simulink model "TrialMBD"  (R2021a)
settings: Solver=FixedStepDiscrete  StartTime=0.0  StopTime=10.0  RelTol=1e-3
libraries: simulink x2
settings Model: Creator=Mahmoud Sofar  LastModifiedBy=Mahmoud Sofar
settings OptimizationCC: DefaultParameterBehavior=Inlined  EnhancedBackFolding=on  PassReuseOutputArgsAs=Individual arguments  ZeroExternalMemoryAtStartup=off  ZeroInternalMemoryAtStartup=off  OptimizeBlockOrder=speed  DifferentSizesBufferReuse=on  OptimizationCustomize=off  EfficientTunableParamExpr=on
settings DebuggingCC: ParameterTunabilityLossMsg=error
settings SFSimCC: MATLABDynamicMemAlloc=off
settings RTWCC: SystemTargetFile=ert.tlc  GenCodeOnly=on  TemplateMakefile=ert_default_tmf  GenerateReport=on  IncludeHyperlinkInReport=on  LaunchReport=on  GenerateTraceInfo=on
settings CodeAppCC: ForceParamTrailComments=on  IgnoreCustomStorageClasses=off  OperatorAnnotations=on  SimulinkDataObjDesc=on  SFDataObjDesc=on  InsertBlockDesc=on
settings ERTTargetCC: TargetLangStandard=C99 (ISO)  GenerateSampleERTMain=on  InlinedParameterPlacement=NonHierarchical  ERTCustomFileTemplate=example_file_process.tlc

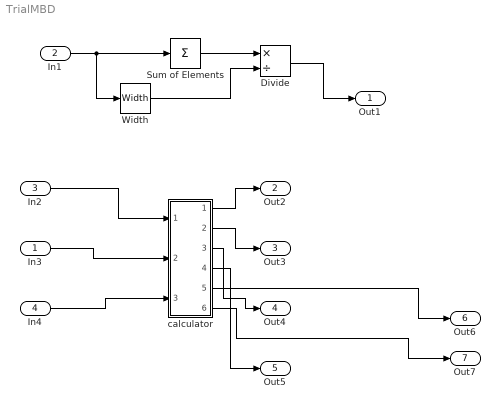
== system TrialMBD ==
  In3 : Inport  PortDimensions=1
  In1 : Inport  Port=2  PortDimensions=11
  In2 : Inport  Port=3  PortDimensions=1
  In4 : Inport  Port=4  PortDimensions=1
  Divide : Product  Inputs=*/
  Sum of Elements : Sum  Inputs=+
  Width : Width
  calculator : Subsystem
  Out1 : Outport
  Out2 : Outport  Port=2
  Out3 : Outport  Port=3
  Out4 : Outport  Port=4
  Out5 : Outport  Port=5
  Out6 : Outport  Port=6
  Out7 : Outport  Port=7
  wires:
  In1/1 -> Width/1, Sum of Elements/1
  Sum of Elements/1 -> Divide/1
  Divide/1 -> Out1/1
  Width/1 -> Divide/2
  In2/1 -> calculator/1(In2)
  In3/1 -> calculator/2(In3)
  In4/1 -> calculator/3(In4)
  calculator/1(Out2) -> Out2/1
  calculator/2(Out3) -> Out3/1
  calculator/3(Out4) -> Out4/1
  calculator/4(Out5) -> Out5/1
  calculator/5(Out6) -> Out6/1
  calculator/6(Out7) -> Out7/1

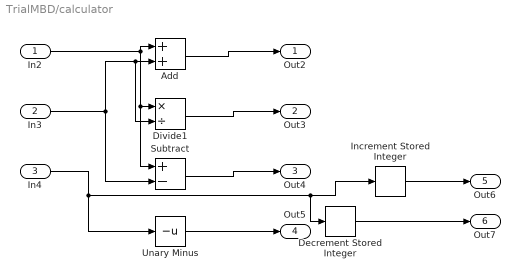
== system TrialMBD/calculator ==
  In2 : Inport  PortDimensions=1
  In3 : Inport  Port=2  PortDimensions=1
  In4 : Inport  Port=3  PortDimensions=1
  Add : Sum
  Decrement Stored Integer : simulink/Additional Math & Discrete/Additional Math: Increment - Decrement/Decrement Stored Integer
      settings: SourceProductBaseCode=SL
  Divide1 : Product  Inputs=*/
  Increment Stored Integer : simulink/Additional Math & Discrete/Additional Math: Increment - Decrement/Increment Stored Integer
  Subtract : Sum  Inputs=+-
  Unary Minus : UnaryMinus
  Out2 : Outport
  Out3 : Outport  Port=2
  Out4 : Outport  Port=3
  Out5 : Outport  Port=4
  Out6 : Outport  Port=5
  Out7 : Outport  Port=6
  wires:
  In4/1 -> Increment Stored Integer/1, Decrement Stored Integer/1, Unary Minus/1
  In3/1 -> Subtract/2, Divide1/2, Add/2
  In2/1 -> Add/1, Divide1/1, Subtract/1
  Decrement Stored Integer/1 -> Out7/1
  Add/1 -> Out2/1
  Increment Stored Integer/1 -> Out6/1
  Subtract/1 -> Out4/1
  Unary Minus/1 -> Out5/1
  Divide1/1 -> Out3/1
